simulink model "Sim27"  (R2019a)
settings: Solver=FixedStepAuto  StartTime=0.0  StopTime=10.0  FixedStep=0.0001  RelTol=1e-3
settings Model: Creator=fbleo  LastModifiedBy=fbleo

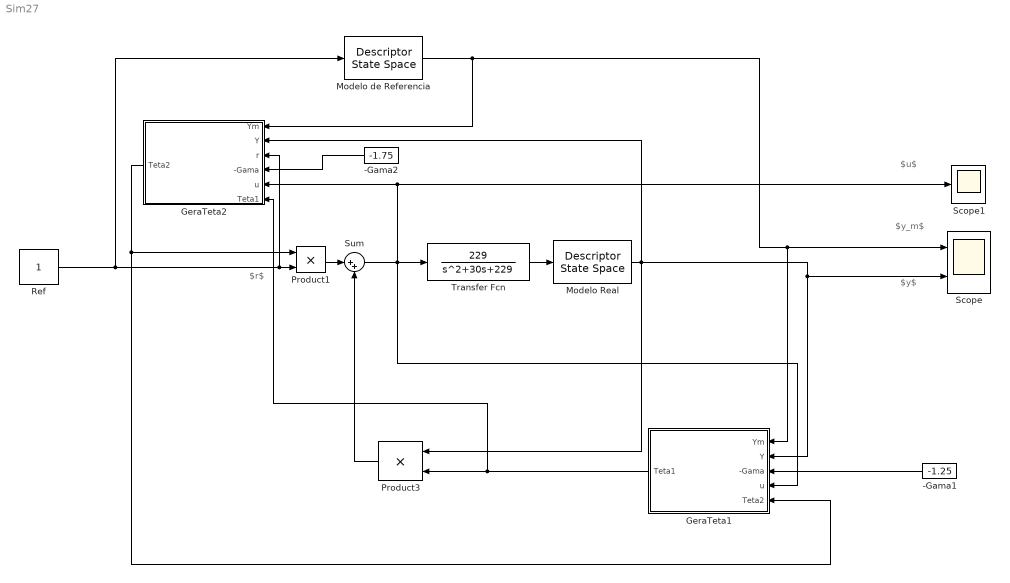
== system Sim27 ==
  note: $r$
  note: $y$
  note: $y_m$
  note: $u$
  -Gama1 : Constant  Value=-1.25
  -Gama2 : Constant  Value=-1.75
  GeraTeta1 : Subsystem
  GeraTeta2 : Subsystem
  Modelo Real : DescriptorStateSpace  A=-1  B=2  D=0  InitialCondition=0.5
  Modelo de Referencia : DescriptorStateSpace  A=-3  B=3  D=0  InitialCondition=0
  Product1 : Product
  Product3 : Product
  Ref : Constant
  Scope : Scope  NumInputPorts=2
  Scope1 : Scope
  Sum : Sum  Inputs=|++
  Transfer Fcn : TransferFcn  Numerator=[229]  Denominator=[1 30 229]
  wires:
  Transfer Fcn/1 -> Modelo Real/1
  Product1/1 -> Sum/1
  Product3/1 -> Sum/2
  -Gama2/1 -> GeraTeta2/4(-Gama)
  Modelo de Referencia/1 -> GeraTeta2/1(Ym), GeraTeta1/1(Ym), Scope/1
  GeraTeta1/1(Teta1) -> GeraTeta2/6("Teta1 "), Product3/2
  -Gama1/1 -> GeraTeta1/3(-Gama)
  Ref/1 -> GeraTeta2/3(r), Product1/2, Modelo de Referencia/1
  GeraTeta2/1(Teta2) -> GeraTeta1/5("Teta2 "), Product1/1
  Modelo Real/1 -> GeraTeta2/2(Y), GeraTeta1/2(Y), Scope/2, Product3/1
  Sum/1 -> GeraTeta1/4(u), Scope1/1, GeraTeta2/5(u), Transfer Fcn/1

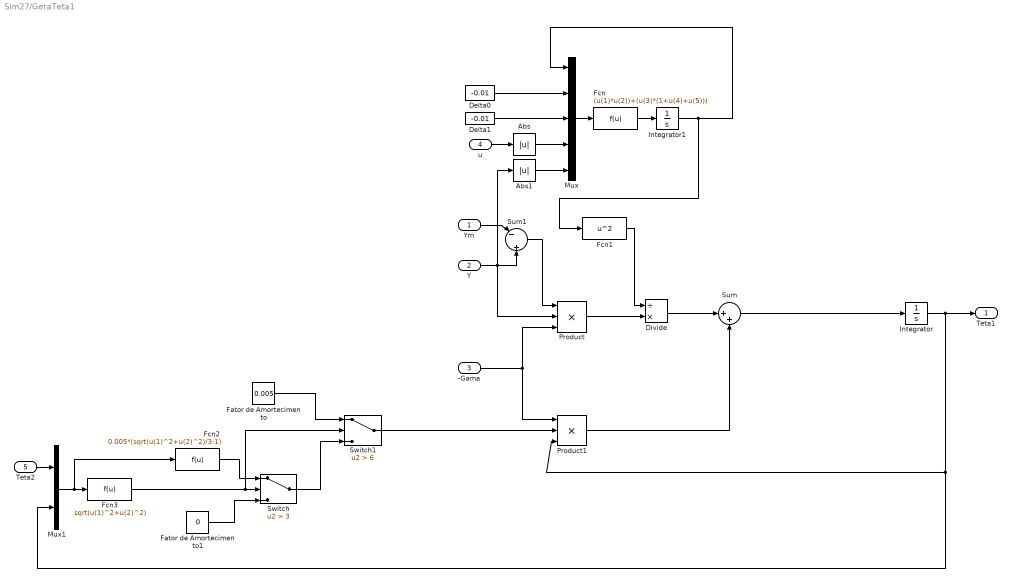
== system Sim27/GeraTeta1 ==
  Ym : Inport
  Y : Inport  Port=2
  -Gama : Inport  Port=3
  u : Inport  Port=4
  "Teta2 " : Inport  Port=5
  Abs : Abs
  Abs1 : Abs
  Delta0 : Constant  Value=-0.01
  Delta1 : Constant  Value=-0.01
  Divide : Product  Inputs=/*
  Fator de Amortecimento : Constant  Value=0.005
  Fator de Amortecimento1 : Constant  Value=0
  Fcn : Fcn  Expr=(u(1)*u(2))+(u(3)*(1+u(4)+u(5)))
  Fcn1 : Fcn  Expr=u^2
  Fcn2 : Fcn  Expr=0.005*(sqrt(u(1)^2+u(2)^2)/3-1)
  Fcn3 : Fcn  Expr=sqrt(u(1)^2+u(2)^2)
  Integrator : Integrator  InitialCondition=-0.65
  Integrator1 : Integrator  InitialCondition=1.1
  Mux : Mux  Inputs=5
  Mux1 : Mux  Inputs=2
  Product : Product  Inputs=3
  Product1 : Product  Inputs=3
  Sum : Sum  Inputs=|++
  Sum1 : Sum  Inputs=|-||+
  Switch : Switch  Criteria=u2 > Threshold  Threshold=3
  Switch1 : Switch  Criteria=u2 > Threshold  Threshold=6
  Teta1 : Outport
  wires:
  Ym/1 -> Sum1/1
  Sum1/1 -> Product/1
  Y/1 -> Product/2, Abs1/1, Sum1/2
  -Gama/1 -> Product1/1, Product/3
  Integrator/1 -> Mux1/2, Product1/3, Teta1/1
  Sum/1 -> Integrator/1
  Product1/1 -> Sum/2
  Product/1 -> Divide/2
  Divide/1 -> Sum/1
  Mux/1 -> Fcn/1
  Fcn/1 -> Integrator1/1
  Delta0/1 -> Mux/2
  Delta1/1 -> Mux/3
  u/1 -> Abs/1
  Abs/1 -> Mux/4
  Abs1/1 -> Mux/5
  Integrator1/1 -> Fcn1/1, Mux/1
  Fcn1/1 -> Divide/1
  Fcn2/1 -> Switch/1
  Fator de Amortecimento1/1 -> Switch/3
  Switch/1 -> Switch1/3
  "Teta2 "/1 -> Mux1/1
  Mux1/1 -> Fcn2/1, Fcn3/1
  Fcn3/1 -> Switch1/2, Switch/2
  Fator de Amortecimento/1 -> Switch1/1
  Switch1/1 -> Product1/2

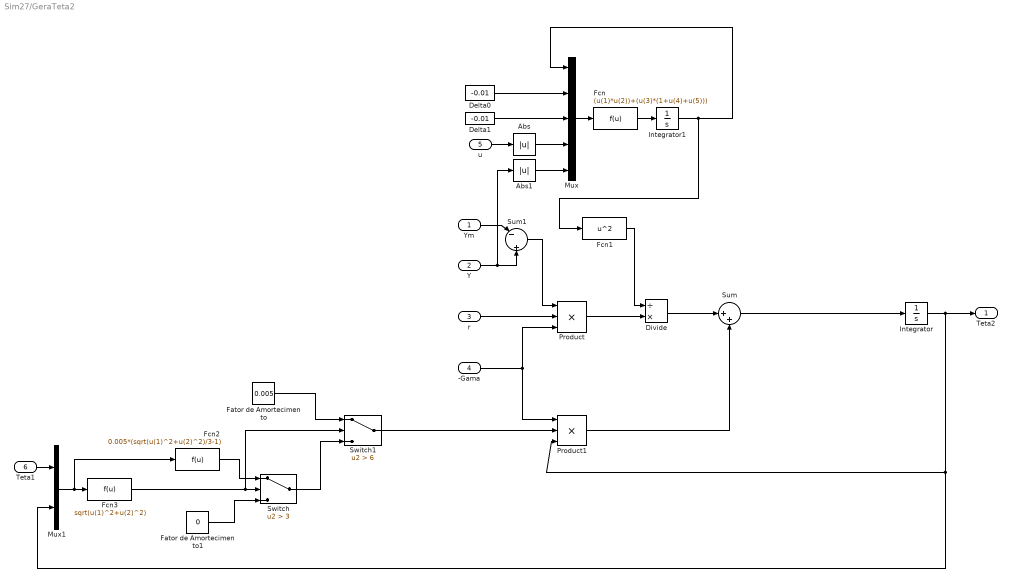
== system Sim27/GeraTeta2 ==
  Ym : Inport
  Y : Inport  Port=2
  r : Inport  Port=3
  -Gama : Inport  Port=4
  u : Inport  Port=5
  "Teta1 " : Inport  Port=6
  Abs : Abs
  Abs1 : Abs
  Delta0 : Constant  Value=-0.01
  Delta1 : Constant  Value=-0.01
  Divide : Product  Inputs=/*
  Fator de Amortecimento : Constant  Value=0.005
  Fator de Amortecimento1 : Constant  Value=0
  Fcn : Fcn  Expr=(u(1)*u(2))+(u(3)*(1+u(4)+u(5)))
  Fcn1 : Fcn  Expr=u^2
  Fcn2 : Fcn  Expr=0.005*(sqrt(u(1)^2+u(2)^2)/3-1)
  Fcn3 : Fcn  Expr=sqrt(u(1)^2+u(2)^2)
  Integrator : Integrator  InitialCondition=1.14
  Integrator1 : Integrator  InitialCondition=1.1
  Mux : Mux  Inputs=5
  Mux1 : Mux  Inputs=2
  Product : Product  Inputs=3
  Product1 : Product  Inputs=3
  Sum : Sum  Inputs=|++
  Sum1 : Sum  Inputs=|-||+
  Switch : Switch  Criteria=u2 > Threshold  Threshold=3
  Switch1 : Switch  Criteria=u2 > Threshold  Threshold=6
  Teta2 : Outport
  wires:
  Ym/1 -> Sum1/1
  Y/1 -> Abs1/1, Sum1/2
  Sum1/1 -> Product/1
  r/1 -> Product/2
  -Gama/1 -> Product1/1, Product/3
  Integrator/1 -> Mux1/2, Product1/3, Teta2/1
  Sum/1 -> Integrator/1
  Product1/1 -> Sum/2
  Product/1 -> Divide/2
  Divide/1 -> Sum/1
  Mux/1 -> Fcn/1
  Fcn/1 -> Integrator1/1
  Delta0/1 -> Mux/2
  Delta1/1 -> Mux/3
  u/1 -> Abs/1
  Abs/1 -> Mux/4
  Abs1/1 -> Mux/5
  Integrator1/1 -> Fcn1/1, Mux/1
  Fcn1/1 -> Divide/1
  Fcn2/1 -> Switch/1
  Fator de Amortecimento1/1 -> Switch/3
  Switch/1 -> Switch1/3
  "Teta1 "/1 -> Mux1/1
  Mux1/1 -> Fcn2/1, Fcn3/1
  Fcn3/1 -> Switch1/2, Switch/2
  Fator de Amortecimento/1 -> Switch1/1
  Switch1/1 -> Product1/2
